simulink model "chap5_13sim"  (Simulink 7.7)
settings: Solver=ode45  StartTime=0.0  StopTime=100  FixedStep=0.001  RelTol=1e-3  AbsTol=1e-3
settings Model: Creator=ljk  LastModifiedBy=ljk  ExtModeTrigMode=oneshot  ExtModeArmWhenConnect=off
settings DataIOCC: LimitDataPoints=off  SignalLoggingName=sigsOut
settings OptimizationCC: BooleanDataType=off  InitFltsAndDblsToZero=on
settings DebuggingCC: SaveWithParameterizedLinksMsg=none  SignalResolutionControl=TryResolveAllWithWarning  SolverPrmCheckMsg=none  MultiTaskDSMMsg=warning  MultiTaskCondExecSysMsg=none  StrictBusMsg=None
settings HardwareCC: TargetUnknown=on
settings RTWCC: IncludeERTFirstTime=on
settings GRTTargetCC: TargetFcnLib=ansi_tfl_tmw.mat

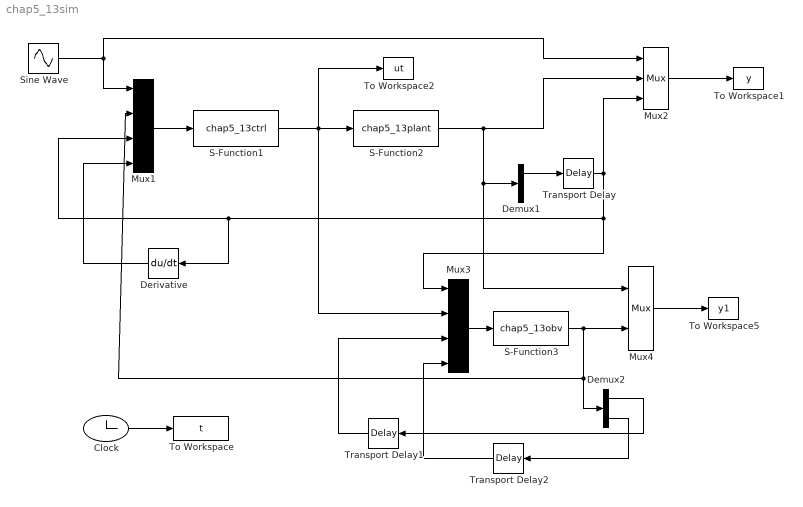
== system chap5_13sim ==
  Clock : Clock
  Demux1 : Demux  Outputs=2
  Demux2 : Demux  Outputs=2
  Derivative : Derivative
  Mux1 : Mux
  Mux2 : Mux  Inputs=3
  Mux3 : Mux
  Mux4 : Mux  Inputs=2
  S-Function1 : S-Function  FunctionName=chap5_13ctrl  EnableBusSupport=off
  S-Function2 : S-Function  FunctionName=chap5_13plant  EnableBusSupport=off
  S-Function3 : S-Function  FunctionName=chap5_13obv  EnableBusSupport=off
  Sine Wave : Sin  SampleTime=0
  To Workspace : ToWorkspace  VariableName=t  SampleTime=-1  SaveFormat=Array
  To Workspace1 : ToWorkspace  VariableName=y  SampleTime=-1  SaveFormat=Array
  To Workspace2 : ToWorkspace  VariableName=ut  SampleTime=-1  SaveFormat=Array
  To Workspace5 : ToWorkspace  VariableName=y1  SampleTime=-1  SaveFormat=Array
  Transport Delay : TransportDelay  DelayTime=3
  Transport Delay1 : TransportDelay  DelayTime=3
  Transport Delay2 : TransportDelay  DelayTime=3
  wires:
  Clock/1 -> To Workspace/1
  Mux3/1 -> S-Function3/1
  Sine Wave/1 -> Mux1/1, Mux2/1
  S-Function2/1 -> Demux1/1, Mux4/1, Mux2/2
  Demux1/1 -> Transport Delay/1
  Transport Delay/1 -> Mux3/1, Mux1/3, Derivative/1, Mux2/3
  Mux2/1 -> To Workspace1/1
  Mux4/1 -> To Workspace5/1
  S-Function3/1 -> Mux4/2, Demux2/1, Mux1/2
  Demux2/1 -> Transport Delay1/1
  Demux2/2 -> Transport Delay2/1
  Transport Delay1/1 -> Mux3/3
  Transport Delay2/1 -> Mux3/4
  Derivative/1 -> Mux1/4
  S-Function1/1 -> S-Function2/1, Mux3/2, To Workspace2/1
  Mux1/1 -> S-Function1/1
